simulink model "rocket_nozzle_acausal_thermal_simulation"  (R2022b)
settings: Solver=ode15s  StartTime=ti(1)  StopTime=ti(3)  RelTol=RelTol  AbsTol=AbsTol
values from neighbouring files (symbols this model uses):
  m2 = S*l(2)*rho2    [rocket_nozzle_causal_thermal_simulation.m]
  m4 = S*l(4)*rho4    [rocket_nozzle_causal_thermal_simulation.m]
  R = l./(S*k)    [rocket_nozzle_causal_thermal_simulation.m]
  T0 = 20+273.15    (= 293.15)    [rocket_nozzle_causal_thermal_simulation.m]
  Tf = 1000+273.15    (= 1273.15)    [rocket_nozzle_causal_thermal_simulation.m]
  ti = [0 1 60]    [rocket_nozzle_causal_thermal_simulation.m]
libraries: fl_lib x46, nesl_utility x14, simulink x2
settings Model: Creator=mutti  LastModifiedBy=mutti
settings SolverCC: AutoScaleAbsTol=off  AlgebraicLoopSolver=TrustRegion  MaxZcPerStep=1
settings DebuggingCC: UnconnectedInputMsg=warning  UnconnectedOutputMsg=warning  UnconnectedLineMsg=warning  SymbolicDimsDataTypeCodeGenerationDiagnostic=none  SFMachineParentedDataDiag=warning
settings ModelReferenceCC: EnableRefExpFcnMdlSchedulingChecks=on
settings SFSimCC: CustomCodeUndefinedFunction=UseInterfaceOnly
settings RTWCC: DLArmComputeVersion=19.05
settings SimscapeCC: SimscapeLogType=all  SimscapeLogSimulationStatistics=on  SimscapeLogDataHistory=10000

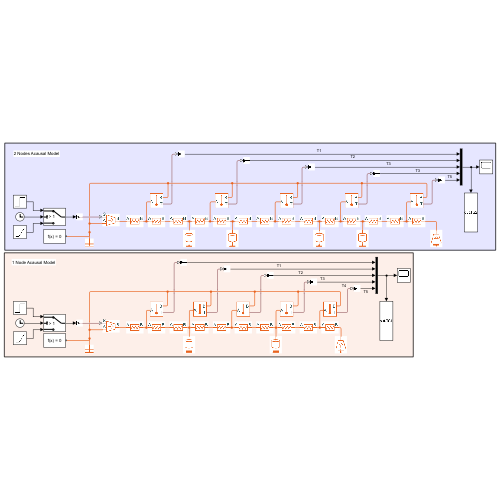
[thumbnail: Simulink's stored preview of the top-level diagram]
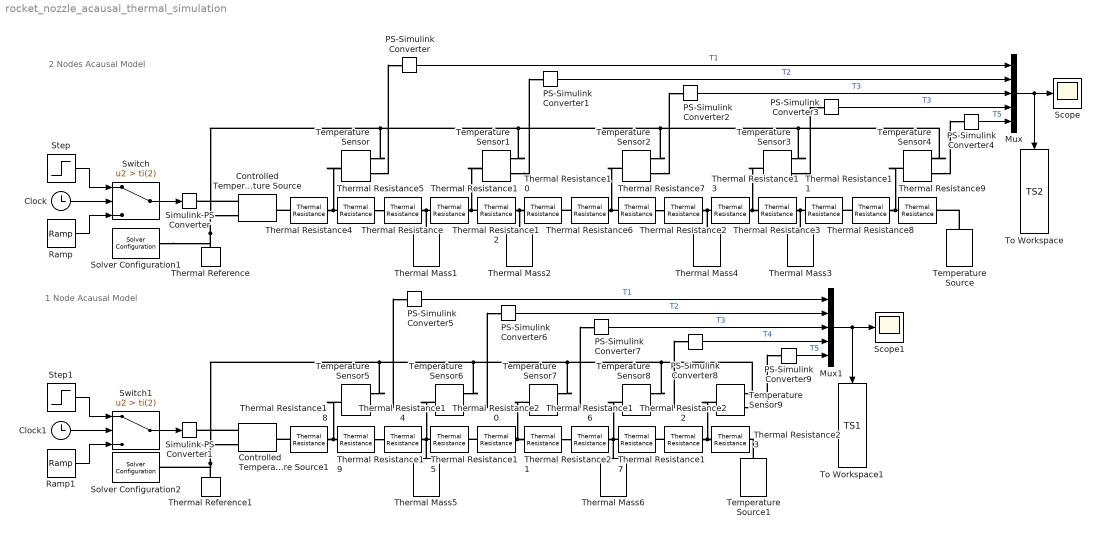
== system rocket_nozzle_acausal_thermal_simulation ==
  note: 1 Node Acausal Model
  note: 2 Nodes Acausal Model
  Clock : Clock
  Clock1 : Clock
  Controlled Temperature Source : fl_lib/Thermal/Thermal Sources/Controlled Temperature Source
  Controlled Temperature Source1 : fl_lib/Thermal/Thermal Sources/Controlled Temperature Source
  Mux : Mux  Inputs=5
  Mux1 : Mux  Inputs=5
  PS-Simulink Converter{,1..9} (10 alike) : nesl_utility/PS-Simulink Converter  PhysicalDomain=network_engine_domain  SubClassName=ps_output  LeftPortType=input  RightPortType=output  PseudoPeriodic=off  Frequencies=[]  VectorFormat=inherit  Unit=inherit  AffineConversion=off
  Ramp : simulink/Sources/Ramp  slope=(Tf-T0)/(ti(2)-ti(1))  start=ti(1)  InitialOutput=T0
  Ramp1 : simulink/Sources/Ramp  slope=(Tf-T0)/(ti(2)-ti(1))  start=ti(1)  InitialOutput=T0
  Scope : Scope
  Scope1 : Scope
  Simulink-PS Converter : nesl_utility/Simulink-PS Converter  PhysicalDomain=network_engine_domain  SubClassName=ps_input  LeftPortType=input  RightPortType=output  PseudoPeriodic=off  Frequencies=[]  NoiseDistribution=none  NoiseParameters=[]  Unit=1  AffineConversion=off  FilteringAndDerivatives=provide  SimscapeFilterOrder=1  InputFilterTimeConstant=0.001  UdotUserProvided=0
  Simulink-PS Converter1 : nesl_utility/Simulink-PS Converter  PhysicalDomain=network_engine_domain  SubClassName=ps_input  LeftPortType=input  RightPortType=output  PseudoPeriodic=off  Frequencies=[]  NoiseDistribution=none  NoiseParameters=[]  Unit=1  AffineConversion=off  FilteringAndDerivatives=provide  SimscapeFilterOrder=1  InputFilterTimeConstant=0.001  UdotUserProvided=0
  Solver Configuration1 : nesl_utility/Solver Configuration  PhysicalDomain=network_engine_domain  SubClassName=solver  LeftPortType=input  RightPortType=generic  Tones=[]  Harmonics=[]  SimulateNoise=off  Profile=off  UseLocalSampling=off  EnableSwitchedLinearOptims=on  FrequencyDomain=off  UseCCode=off  RelTol=0.001  AbsTol=0.001  MinStep=1e-09  ToWorkspace=off  RevertToSquareIcSolve=off  NumHomotopyIterations=100  PhasorMode=off  PhasorModeNumHarmonics=1  ConsistencySolver=NEWTON_XTOL_AFTER_FTOL  IndexReductionMethod=DerivativeReplacement  DoDC=off  ResidualTolerance=1e-09  ConsistencyTolSource=GLOBAL  ConsistencyAbsTol=0.001  ConsistencyRelTol=0.001  ConsistencyTolFactor=0.001  UseLocalSolver=off  LocalSolverChoice=NE_BACKWARD_EULER_ADVANCER  ResolveIndetEquations=on  FunctionEvalNumThread=1  LocalSolverSampleTime=0.001  DoFixedCost=off  MaxNonlinIter=3  MaxModeIter=2  ComputeImpulses=off  ImpulseIterations=2  LinearAlgebra=auto  LinearAlgebraNumThread=0  EquationFormulation=NE_TIME_EF  DelaysMemoryBudget=1024  AutomaticFiltering=on  FilteringTimeConstant=0.001  PartitionStorageMethod=AS_NEEDED  PartitionMemoryBudget=1024  PartitionMethod=ROBUST
  Solver Configuration2 : nesl_utility/Solver Configuration  PhysicalDomain=network_engine_domain  SubClassName=solver  LeftPortType=input  RightPortType=generic  Tones=[]  Harmonics=[]  SimulateNoise=off  Profile=off  UseLocalSampling=off  EnableSwitchedLinearOptims=on  FrequencyDomain=off  UseCCode=off  RelTol=0.001  AbsTol=0.001  MinStep=1e-09  ToWorkspace=off  RevertToSquareIcSolve=off  NumHomotopyIterations=100  PhasorMode=off  PhasorModeNumHarmonics=1  ConsistencySolver=NEWTON_XTOL_AFTER_FTOL  IndexReductionMethod=DerivativeReplacement  DoDC=off  ResidualTolerance=1e-09  ConsistencyTolSource=GLOBAL  ConsistencyAbsTol=0.001  ConsistencyRelTol=0.001  ConsistencyTolFactor=0.001  UseLocalSolver=off  LocalSolverChoice=NE_BACKWARD_EULER_ADVANCER  ResolveIndetEquations=on  FunctionEvalNumThread=1  LocalSolverSampleTime=0.001  DoFixedCost=off  MaxNonlinIter=3  MaxModeIter=2  ComputeImpulses=off  ImpulseIterations=2  LinearAlgebra=auto  LinearAlgebraNumThread=0  EquationFormulation=NE_TIME_EF  DelaysMemoryBudget=1024  AutomaticFiltering=on  FilteringTimeConstant=0.001  PartitionStorageMethod=AS_NEEDED  PartitionMemoryBudget=1024  PartitionMethod=ROBUST
  Step : Step  Time=0  After=Tf  SampleTime=0
  Step1 : Step  Time=0  After=Tf  SampleTime=0
  Switch : Switch  Criteria=u2 > Threshold  Threshold=ti(2)  SaturateOnIntegerOverflow=off  InputSameDT=off
  Switch1 : Switch  Criteria=u2 > Threshold  Threshold=ti(2)  SaturateOnIntegerOverflow=off  InputSameDT=off
  Temperature Sensor{,1..9} (10 alike) : fl_lib/Thermal/Thermal Sensors/Temperature Sensor
  Temperature Source : fl_lib/Thermal/Thermal Sources/Temperature Source  temperature=T0 K
  Temperature Source1 : fl_lib/Thermal/Thermal Sources/Temperature Source  temperature=T0 K
  Thermal Mass1 : fl_lib/Thermal/Thermal Elements/Thermal Mass  mass=m2/2 kg  sp_heat=cp2 J/(K*kg)  num_ports=foundation.enum.numPorts2.one  T_specify=on  T_priority=High  T=T0 K  T_nominal_specify=off  T_nominal_unit=K  T_nominal_value=1  Q_specify=off  Q_priority=None  Q=0 W  Q_nominal_specify=off  Q_nominal_unit=W  Q_nominal_value=1
  Thermal Mass2 : fl_lib/Thermal/Thermal Elements/Thermal Mass  mass=m2/2 kg  sp_heat=cp2 J/(K*kg)  num_ports=foundation.enum.numPorts2.one  T_specify=on  T_priority=High  T=T0 K  T_nominal_specify=off  T_nominal_unit=K  T_nominal_value=1  Q_specify=off  Q_priority=None  Q=0 W  Q_nominal_specify=off  Q_nominal_unit=W  Q_nominal_value=1
  Thermal Mass3 : fl_lib/Thermal/Thermal Elements/Thermal Mass  mass=m4/2 kg  sp_heat=cp4 J/(K*kg)  num_ports=foundation.enum.numPorts2.one  T_specify=on  T_priority=High  T=T0 K  T_nominal_specify=off  T_nominal_unit=K  T_nominal_value=1  Q_specify=off  Q_priority=None  Q=0 W  Q_nominal_specify=off  Q_nominal_unit=W  Q_nominal_value=1
  Thermal Mass4 : fl_lib/Thermal/Thermal Elements/Thermal Mass  mass=m4/2 kg  sp_heat=cp4 J/(K*kg)  num_ports=foundation.enum.numPorts2.one  T_specify=on  T_priority=High  T=T0 K  T_nominal_specify=off  T_nominal_unit=K  T_nominal_value=1  Q_specify=off  Q_priority=None  Q=0 W  Q_nominal_specify=off  Q_nominal_unit=W  Q_nominal_value=1
  Thermal Mass5 : fl_lib/Thermal/Thermal Elements/Thermal Mass  mass=m2 kg  sp_heat=cp2 J/(K*kg)  num_ports=foundation.enum.numPorts2.one  T_specify=on  T_priority=High  T=T0 K  T_nominal_specify=off  T_nominal_unit=K  T_nominal_value=1  Q_specify=off  Q_priority=None  Q=0 W  Q_nominal_specify=off  Q_nominal_unit=W  Q_nominal_value=1
  Thermal Mass6 : fl_lib/Thermal/Thermal Elements/Thermal Mass  mass=m4 kg  sp_heat=cp4 J/(K*kg)  num_ports=foundation.enum.numPorts2.one  T_specify=on  T_priority=High  T=T0 K  T_nominal_specify=off  T_nominal_unit=K  T_nominal_value=1  Q_specify=off  Q_priority=None  Q=0 W  Q_nominal_specify=off  Q_nominal_unit=W  Q_nominal_value=1
  Thermal Reference : fl_lib/Thermal/Thermal Elements/Thermal Reference
  Thermal Reference1 : fl_lib/Thermal/Thermal Elements/Thermal Reference
  Thermal Resistance : fl_lib/Thermal/Thermal Elements/Thermal Resistance  resistance=R(2)/3 K/W  T_specify=on  T_priority=High  T=0 K  T_nominal_specify=off  T_nominal_unit=K  T_nominal_value=1  Q_specify=off  Q_priority=None  Q=0 W  Q_nominal_specify=off  Q_nominal_unit=W  Q_nominal_value=1
  Thermal Resistance1 : fl_lib/Thermal/Thermal Elements/Thermal Resistance  resistance=R(2)/6 K/W  T_specify=on  T_priority=High  T=0 K  T_nominal_specify=off  T_nominal_unit=K  T_nominal_value=1  Q_specify=off  Q_priority=None  Q=0 W  Q_nominal_specify=off  Q_nominal_unit=W  Q_nominal_value=1
  Thermal Resistance10 : fl_lib/Thermal/Thermal Elements/Thermal Resistance  resistance=R(2)/3 K/W  T_specify=on  T_priority=High  T=0 K  T_nominal_specify=off  T_nominal_unit=K  T_nominal_value=1  Q_specify=off  Q_priority=None  Q=0 W  Q_nominal_specify=off  Q_nominal_unit=W  Q_nominal_value=1
  Thermal Resistance11 : fl_lib/Thermal/Thermal Elements/Thermal Resistance  resistance=R(4)/3 K/W  T_specify=on  T_priority=High  T=0 K  T_nominal_specify=off  T_nominal_unit=K  T_nominal_value=1  Q_specify=off  Q_priority=None  Q=0 W  Q_nominal_specify=off  Q_nominal_unit=W  Q_nominal_value=1
  Thermal Resistance12 : fl_lib/Thermal/Thermal Elements/Thermal Resistance  resistance=R(2)/6 K/W  T_specify=on  T_priority=High  T=0 K  T_nominal_specify=off  T_nominal_unit=K  T_nominal_value=1  Q_specify=off  Q_priority=None  Q=0 W  Q_nominal_specify=off  Q_nominal_unit=W  Q_nominal_value=1
  Thermal Resistance13 : fl_lib/Thermal/Thermal Elements/Thermal Resistance  resistance=R(4)/6 K/W  T_specify=on  T_priority=High  T=0 K  T_nominal_specify=off  T_nominal_unit=K  T_nominal_value=1  Q_specify=off  Q_priority=None  Q=0 W  Q_nominal_specify=off  Q_nominal_unit=W  Q_nominal_value=1
  Thermal Resistance14 : fl_lib/Thermal/Thermal Elements/Thermal Resistance  resistance=R(2)/2 K/W  T_specify=on  T_priority=High  T=0 K  T_nominal_specify=off  T_nominal_unit=K  T_nominal_value=1  Q_specify=off  Q_priority=None  Q=0 W  Q_nominal_specify=off  Q_nominal_unit=W  Q_nominal_value=1
  Thermal Resistance15 : fl_lib/Thermal/Thermal Elements/Thermal Resistance  resistance=R(2)/2 K/W  T_specify=on  T_priority=High  T=0 K  T_nominal_specify=off  T_nominal_unit=K  T_nominal_value=1  Q_specify=off  Q_priority=None  Q=0 W  Q_nominal_specify=off  Q_nominal_unit=W  Q_nominal_value=1
  Thermal Resistance16 : fl_lib/Thermal/Thermal Elements/Thermal Resistance  resistance=R(4)/2 K/W  T_specify=on  T_priority=High  T=0 K  T_nominal_specify=off  T_nominal_unit=K  T_nominal_value=1  Q_specify=off  Q_priority=None  Q=0 W  Q_nominal_specify=off  Q_nominal_unit=W  Q_nominal_value=1
  Thermal Resistance17 : fl_lib/Thermal/Thermal Elements/Thermal Resistance  resistance=R(4)/2 K/W  T_specify=on  T_priority=High  T=0 K  T_nominal_specify=off  T_nominal_unit=K  T_nominal_value=1  Q_specify=off  Q_priority=None  Q=0 W  Q_nominal_specify=off  Q_nominal_unit=W  Q_nominal_value=1
  Thermal Resistance{4..5,18..19} (4 alike) : fl_lib/Thermal/Thermal Elements/Thermal Resistance  resistance=R(1)/2 K/W  T_specify=on  T_priority=High  T=0 K  T_nominal_specify=off  T_nominal_unit=K  T_nominal_value=1  Q_specify=off  Q_priority=None  Q=0 W  Q_nominal_specify=off  Q_nominal_unit=W  Q_nominal_value=1
  Thermal Resistance2 : fl_lib/Thermal/Thermal Elements/Thermal Resistance  resistance=R(4)/3 K/W  T_specify=on  T_priority=High  T=0 K  T_nominal_specify=off  T_nominal_unit=K  T_nominal_value=1  Q_specify=off  Q_priority=None  Q=0 W  Q_nominal_specify=off  Q_nominal_unit=W  Q_nominal_value=1
  Thermal Resistance{6..7,20..21} (4 alike) : fl_lib/Thermal/Thermal Elements/Thermal Resistance  resistance=R(3)/2 K/W  T_specify=on  T_priority=High  T=0 K  T_nominal_specify=off  T_nominal_unit=K  T_nominal_value=1  Q_specify=off  Q_priority=None  Q=0 W  Q_nominal_specify=off  Q_nominal_unit=W  Q_nominal_value=1
  Thermal Resistance{8..9,22..23} (4 alike) : fl_lib/Thermal/Thermal Elements/Thermal Resistance  resistance=R(5)/2 K/W  T_specify=on  T_priority=High  T=0 K  T_nominal_specify=off  T_nominal_unit=K  T_nominal_value=1  Q_specify=off  Q_priority=None  Q=0 W  Q_nominal_specify=off  Q_nominal_unit=W  Q_nominal_value=1
  Thermal Resistance3 : fl_lib/Thermal/Thermal Elements/Thermal Resistance  resistance=R(4)/6 K/W  T_specify=on  T_priority=High  T=0 K  T_nominal_specify=off  T_nominal_unit=K  T_nominal_value=1  Q_specify=off  Q_priority=None  Q=0 W  Q_nominal_specify=off  Q_nominal_unit=W  Q_nominal_value=1
  To Workspace : ToWorkspace  VariableName=TS2  SampleTime=-1
      settings: Save2DSignal=2-D array (concatenate along first dimension)
  To Workspace1 : ToWorkspace  VariableName=TS1  SampleTime=-1
      settings: Save2DSignal=2-D array (concatenate along first dimension)
  wires:
  Clock/1 -> Switch/2
  Ramp/1 -> Switch/3
  Step/1 -> Switch/1
  Switch/1 -> Simulink-PS Converter/1
  PS-Simulink Converter4/1 -> Mux/5  "T5"
  PS-Simulink Converter2/1 -> Mux/3  "T3"
  PS-Simulink Converter/1 -> Mux/1  "T1"
  Mux/1 -> To Workspace/1, Scope/1
  PS-Simulink Converter1/1 -> Mux/2  "T2"
  PS-Simulink Converter3/1 -> Mux/4  "T3"
  PS-Simulink Converter6/1 -> Mux1/2  "T2"
  PS-Simulink Converter8/1 -> Mux1/4  "T4"
  PS-Simulink Converter7/1 -> Mux1/3  "T3"
  PS-Simulink Converter9/1 -> Mux1/5  "T5"
  Switch1/1 -> Simulink-PS Converter1/1
  Mux1/1 -> To Workspace1/1, Scope1/1
  PS-Simulink Converter5/1 -> Mux1/1  "T1"
  Clock1/1 -> Switch1/2
  Ramp1/1 -> Switch1/3
  Step1/1 -> Switch1/1
  connections:
  Thermal Resistance5/RConn1 -- Thermal Resistance/LConn1
  Thermal Mass1/LConn1 -- Thermal Resistance1/LConn1 -- Thermal Resistance/RConn1
  Thermal Mass4/LConn1 -- Thermal Resistance13/LConn1 -- Thermal Resistance2/RConn1
  Thermal Resistance7/RConn1 -- Thermal Resistance2/LConn1
  Thermal Resistance5/LConn1 -- Temperature Sensor/LConn1 -- Thermal Resistance4/RConn1
  Thermal Resistance7/LConn1 -- Temperature Sensor2/LConn1 -- Thermal Resistance6/RConn1
  Thermal Resistance9/LConn1 -- Temperature Sensor4/LConn1 -- Thermal Resistance8/RConn1
  Controlled Temperature Source/RConn1 -- Simulink-PS Converter/RConn1
  Temperature Sensor/RConn1 -- Temperature Sensor4/RConn1 -- Temperature Sensor3/RConn1 -- Temperature Sensor2/RConn1 -- Temperature Sensor1/RConn1 -- Solver Configuration1/RConn1 -- Thermal Reference/LConn1 -- Controlled Temperature Source/RConn2
  Thermal Resistance4/LConn1 -- Controlled Temperature Source/LConn1
  Temperature Sensor/RConn2 -- PS-Simulink Converter/LConn1
  Temperature Sensor2/RConn2 -- PS-Simulink Converter2/LConn1
  Temperature Sensor4/RConn2 -- PS-Simulink Converter4/LConn1
  Temperature Source/LConn1 -- Thermal Resistance9/RConn1
  Thermal Resistance10/LConn1 -- Thermal Resistance12/RConn1 -- Thermal Mass2/LConn1
  Thermal Resistance6/LConn1 -- Thermal Resistance10/RConn1
  Thermal Resistance11/LConn1 -- Thermal Mass3/LConn1 -- Thermal Resistance3/RConn1
  Thermal Resistance8/LConn1 -- Thermal Resistance11/RConn1
  Thermal Resistance12/LConn1 -- Temperature Sensor1/LConn1 -- Thermal Resistance1/RConn1
  Thermal Resistance13/RConn1 -- Temperature Sensor3/LConn1 -- Thermal Resistance3/LConn1
  Temperature Sensor1/RConn2 -- PS-Simulink Converter1/LConn1
  Temperature Sensor3/RConn2 -- PS-Simulink Converter3/LConn1
  Temperature Sensor7/RConn1 -- Temperature Sensor5/RConn1 -- Solver Configuration2/RConn1 -- Thermal Reference1/LConn1 -- Controlled Temperature Source1/RConn2 -- Temperature Sensor6/RConn1 -- Temperature Sensor9/RConn1 -- Temperature Sensor8/RConn1
  Thermal Resistance20/RConn1 -- Thermal Resistance21/LConn1 -- Temperature Sensor7/LConn1
  Thermal Resistance18/RConn1 -- Thermal Resistance19/LConn1 -- Temperature Sensor5/LConn1
  Thermal Resistance17/LConn1 -- Thermal Resistance16/RConn1 -- Thermal Mass6/LConn1 -- Temperature Sensor8/LConn1
  Thermal Resistance22/RConn1 -- Thermal Resistance23/LConn1 -- Temperature Sensor9/LConn1
  Thermal Resistance15/LConn1 -- Thermal Mass5/LConn1 -- Temperature Sensor6/LConn1 -- Thermal Resistance14/RConn1
  Thermal Resistance18/LConn1 -- Controlled Temperature Source1/LConn1
  Thermal Resistance19/RConn1 -- Thermal Resistance14/LConn1
  Controlled Temperature Source1/RConn1 -- Simulink-PS Converter1/RConn1
  Temperature Sensor9/RConn2 -- PS-Simulink Converter9/LConn1
  Temperature Sensor7/RConn2 -- PS-Simulink Converter7/LConn1
  Thermal Resistance21/RConn1 -- Thermal Resistance16/LConn1
  Thermal Resistance22/LConn1 -- Thermal Resistance17/RConn1
  Temperature Sensor6/RConn2 -- PS-Simulink Converter6/LConn1
  Temperature Sensor8/RConn2 -- PS-Simulink Converter8/LConn1
  Temperature Sensor5/RConn2 -- PS-Simulink Converter5/LConn1
  Thermal Resistance20/LConn1 -- Thermal Resistance15/RConn1
  Temperature Source1/LConn1 -- Thermal Resistance23/RConn1
